simulink model "Csim"  (R2016b)
settings: Solver=ode45  StartTime=0.0  StopTime=0.5  RelTol=1e-3
settings Model: Creator=jonathankirchman  LastModifiedBy=jonathankirchman

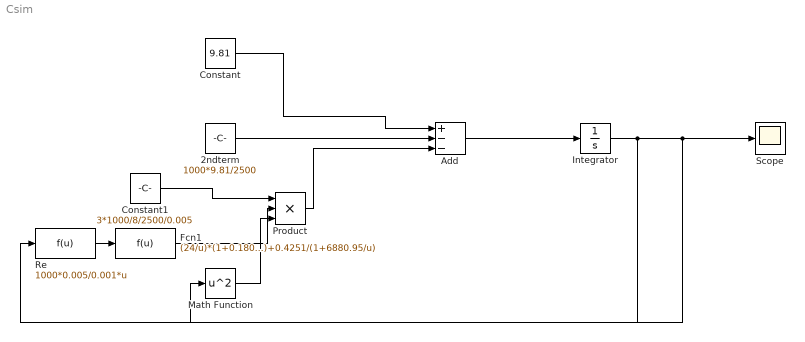
== system Csim ==
  "2ndterm " : Constant  Value=1000*9.81/2500
  Add : Sum  Inputs=+--
  Constant : Constant  Value=9.81
  Constant1 : Constant  Value=3*1000/8/2500/0.005
  Fcn1 : Fcn  Expr=(24/u)*(1+0.18006*u^(0.6459))+0.4251/(1+6880.95/u)
  Integrator : Integrator  InitialCondition=1e-5
  Math Function : Math  Operator=square  SaturateOnIntegerOverflow=on
  Product : Product  Inputs=3
  Re : Fcn  Expr=1000*0.005/0.001*u
  Scope : Scope
  wires:
  Constant/1 -> Add/1
  "2ndterm "/1 -> Add/2
  Constant1/1 -> Product/1
  Math Function/1 -> Product/3
  Re/1 -> Fcn1/1
  Integrator/1 -> Math Function/1, Re/1, Scope/1
  Fcn1/1 -> Product/2
  Product/1 -> Add/3
  Add/1 -> Integrator/1
